simulink model "model"  (R2018b)
settings: Solver=VariableStepAuto  StartTime=0.0  StopTime=10.0  RelTol=1e-2
values from neighbouring files (symbols this model uses):
  alfa = in(2)    [optymalizacja.m]    (also in zawieszenie_dane.m = opti(1))
  beta = in(3)    [optymalizacja.m]    (also in zawieszenie_dane.m = opti(2))
  cc = 15000    [zawieszenie_dane.m]
  cw = 200000    [zawieszenie_dane.m]
  dc = 200    [zawieszenie_dane.m]
  dw = 10    [zawieszenie_dane.m]
  k = in(1)    [optymalizacja.m]    (also in zawieszenie_dane.m = opti(3))
  mc = 250    [zawieszenie_dane.m]
  mw = 30    [zawieszenie_dane.m]
settings Model: Creator=lpa2  LastModifiedBy=Kasia
settings SolverCC: MaxConsecutiveMinStep=100
settings SFSimCC: SimUseLocalCustomCode=off
settings RTWCC: RTWUseLocalCustomCode=off

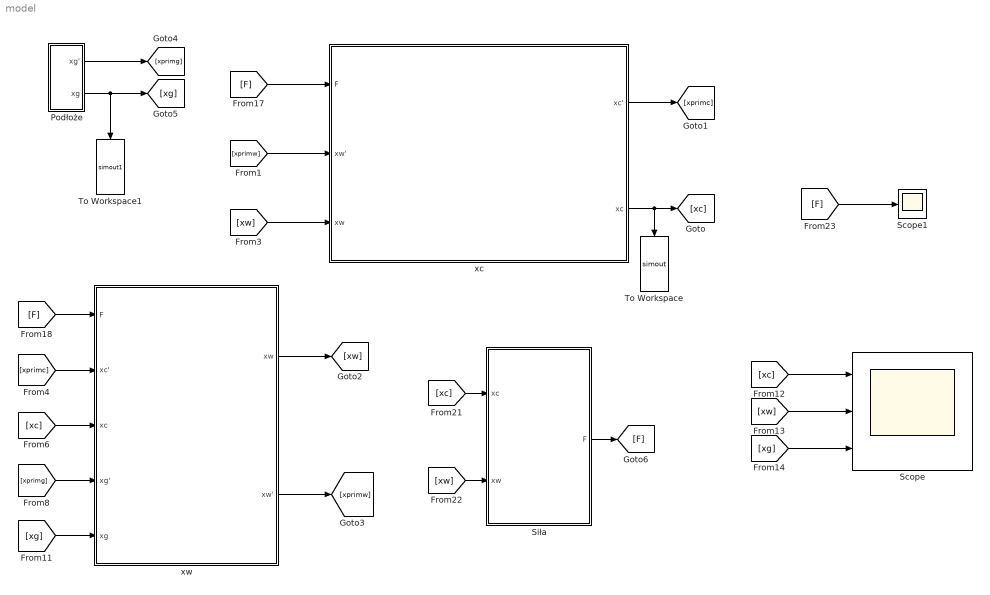
== system model ==
  Podłoże : Subsystem
  Scope : Scope  NumInputPorts=3
  Scope1 : Scope
  Siła : Subsystem
  To Workspace : ToWorkspace  VariableName=simout  SaveFormat=Timeseries  SampleTime=-1
  To Workspace1 : ToWorkspace  VariableName=simout1  SaveFormat=Timeseries  SampleTime=-1
  xc : Subsystem
  xw : Subsystem
  wires:
  [xc] -> Scope/1
  [xw] -> Scope/2
  [xg] -> Scope/3
  [F] -> Scope1/1
  xc/2("xc ") -> [xc], To Workspace/1
  xc/1("xc' ") -> [xprimc]
  [F] -> xc/1(F)
  [xprimw] -> xc/2(xw')
  [xw] -> xc/3("xw ")
  xw/2(xw') -> [xprimw]
  xw/1(xw) -> [xw]
  [F] -> xw/1(F)
  [xprimc] -> xw/2(xc')
  [xc] -> xw/3("xc ")
  [xprimg] -> xw/4(xg')
  [xg] -> xw/5(xg)
  Podłoże/1(xg') -> [xprimg]
  Podłoże/2(xg) -> [xg], To Workspace1/1
  Siła/1("F ") -> [F]
  [xc] -> Siła/1(xc)
  [xw] -> Siła/2(xw)

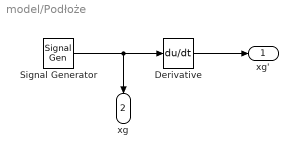
== system model/Podłoże ==
  Derivative : Derivative
  Signal Generator : SignalGenerator  WaveForm=square  Amplitude=0.05  Frequency=0.5  Units=rad/sec
  xg' : Outport
  xg : Outport  Port=2
  wires:
  Derivative/1 -> xg'/1
  Signal Generator/1 -> xg/1, Derivative/1

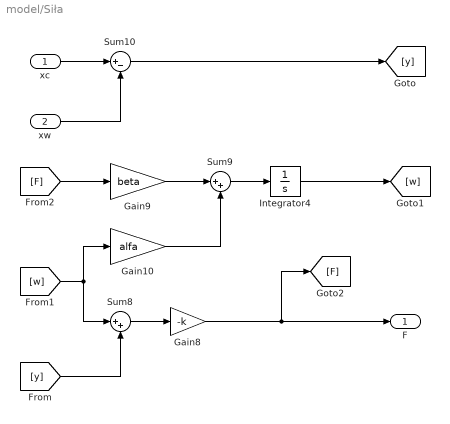
== system model/Siła ==
  xc : Inport
  xw : Inport  Port=2
  Gain10 : Gain  Gain=alfa
  Gain8 : Gain  Gain=-k
  Gain9 : Gain  Gain=beta
  Integrator4 : Integrator
  Sum10 : Sum  Inputs=|+-
  Sum8 : Sum  Inputs=|++
  Sum9 : Sum  Inputs=|++
  "F " : Outport
  wires:
  [w] -> Gain10/1, Sum8/1
  xc/1 -> Sum10/1
  Sum9/1 -> Integrator4/1
  xw/1 -> Sum10/2
  Integrator4/1 -> [w]
  Sum10/1 -> [y]
  Gain10/1 -> Sum9/2
  Sum8/1 -> Gain8/1
  [y] -> Sum8/2
  Gain8/1 -> [F], "F "/1
  [F] -> Gain9/1
  Gain9/1 -> Sum9/1

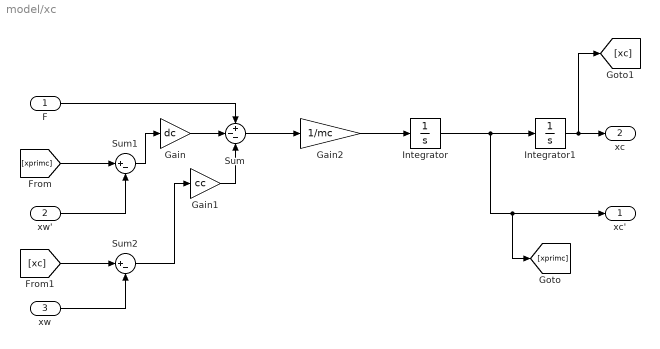
== system model/xc ==
  F : Inport
  xw' : Inport  Port=2
  "xw " : Inport  Port=3
  Gain : Gain  Gain=dc
  Gain1 : Gain  Gain=cc
  Gain2 : Gain  Gain=1/mc
  Integrator : Integrator
  Integrator1 : Integrator
  Sum : Sum  Inputs=+--
  Sum1 : Sum  Inputs=|+-
  Sum2 : Sum  Inputs=|+-
  "xc' " : Outport
  "xc " : Outport  Port=2
  wires:
  Gain/1 -> Sum/2
  Gain1/1 -> Sum/3
  Gain2/1 -> Integrator/1
  [xprimc] -> Sum1/1
  Sum1/1 -> Gain/1
  xw'/1 -> Sum1/2
  Integrator/1 -> [xprimc], "xc' "/1, Integrator1/1
  Sum/1 -> Gain2/1
  [xc] -> Sum2/1
  Sum2/1 -> Gain1/1
  Integrator1/1 -> [xc], "xc "/1
  "xw "/1 -> Sum2/2
  F/1 -> Sum/1

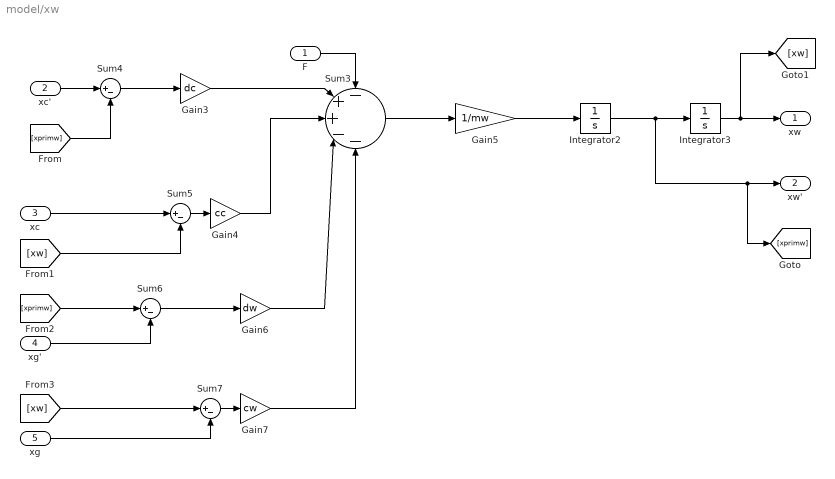
== system model/xw ==
  F : Inport
  xc' : Inport  Port=2
  "xc " : Inport  Port=3
  xg' : Inport  Port=4
  xg : Inport  Port=5
  Gain3 : Gain  Gain=dc
  Gain4 : Gain  Gain=cc
  Gain5 : Gain  Gain=1/mw
  Gain6 : Gain  Gain=dw
  Gain7 : Gain  Gain=cw
  Integrator2 : Integrator
  Integrator3 : Integrator
  Sum3 : Sum  Inputs=-++--
  Sum{4..7} (4 alike) : Sum  Inputs=|+-
  xw : Outport
  xw' : Outport  Port=2
  wires:
  Sum3/1 -> Gain5/1
  Sum4/1 -> Gain3/1
  Gain3/1 -> Sum3/2
  Integrator3/1 -> [xw], xw/1
  [xprimw] -> Sum4/2
  Gain7/1 -> Sum3/5
  Sum7/1 -> Gain7/1
  xg'/1 -> Sum6/2
  F/1 -> Sum3/1
  Gain6/1 -> Sum3/4
  "xc "/1 -> Sum5/1
  Gain5/1 -> Integrator2/1
  Sum6/1 -> Gain6/1
  [xw] -> Sum5/2
  Integrator2/1 -> [xprimw], xw'/1, Integrator3/1
  xc'/1 -> Sum4/1
  Sum5/1 -> Gain4/1
  xg/1 -> Sum7/2
  Gain4/1 -> Sum3/3
  [xprimw] -> Sum6/1
  [xw] -> Sum7/1
